simulink model "SimulacionCTRL3deposicion"  (R2021b)
settings: Solver=VariableStepAuto  StartTime=0.0  StopTime=20  RelTol=1e-3
undefined symbols (not defined in the file): coefDen, coefNum, kdr, ki, ki2, kp, kpr
libraries: simulink x1
settings Model: Creator=nicol  LastModifiedBy=CASA

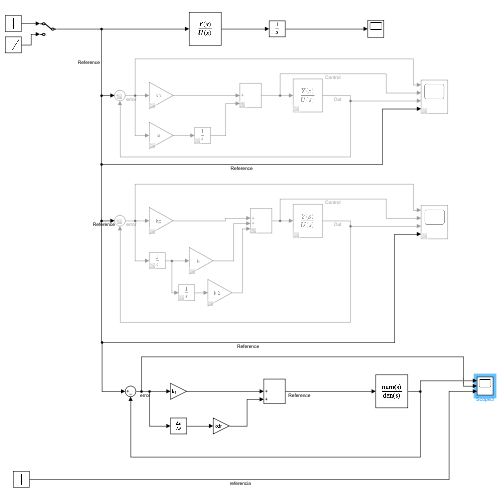
[thumbnail: Simulink's stored preview of the top-level diagram]
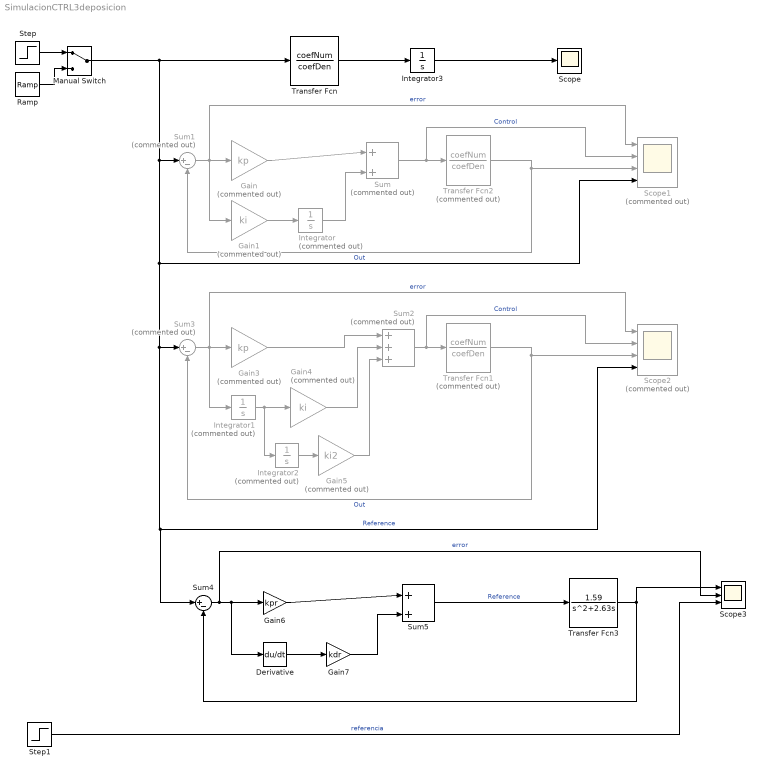
== system SimulacionCTRL3deposicion ==
  Derivative : Derivative
  Gain : Gain  Commented=on  Gain=kp
  Gain1 : Gain  Commented=on  Gain=ki
  Gain3 : Gain  Commented=on  Gain=kp
  Gain4 : Gain  Commented=on  Gain=ki
  Gain5 : Gain  Commented=on  Gain=ki2
  Gain6 : Gain  Gain=kpr
  Gain7 : Gain  Gain=kdr
  Integrator : Integrator  Commented=on
  Integrator1 : Integrator  Commented=on
  Integrator2 : Integrator  Commented=on
  Integrator3 : Integrator
  Manual Switch : ManualSwitch
  Ramp : simulink/Sources/Ramp  slope=1  start=0  InitialOutput=0
  Scope : Scope
  Scope1 : Scope  Commented=on  NumInputPorts=4
  Scope2 : Scope  Commented=on  NumInputPorts=4
  Scope3 : Scope  NumInputPorts=3
  Step : Step  Time=0  SampleTime=0
  Step1 : Step  Time=0  SampleTime=0
  Sum : Sum  Commented=on  Inputs=|++
  Sum1 : Sum  Commented=on  Inputs=|+-
  Sum2 : Sum  Commented=on  Inputs=|+++
  Sum3 : Sum  Commented=on  Inputs=|+-
  Sum4 : Sum  Inputs=|+-
  Sum5 : Sum  Inputs=|++
  Transfer Fcn : TransferFcn  Numerator=coefNum  Denominator=coefDen
  Transfer Fcn1 : TransferFcn  Commented=on  Numerator=coefNum  Denominator=coefDen
  Transfer Fcn2 : TransferFcn  Commented=on  Numerator=coefNum  Denominator=coefDen
  Transfer Fcn3 : TransferFcn  Numerator=[1.59]  Denominator=[1 2.63 0]
  wires:
  Gain1/1 -> Integrator/1
  Gain/1 -> Sum/1
  Integrator/1 -> Sum/2
  Sum/1 -> Scope1/2, Transfer Fcn2/1  "Control"
  Sum1/1 -> Gain1/1, Scope1/1, Gain/1  "error"
  Transfer Fcn2/1 -> Scope1/3, Sum1/2  "Out"
  Manual Switch/1 -> Sum3/1, Sum4/1, Scope2/4, Scope1/4, Sum1/1, Transfer Fcn/1  "Reference"
  Transfer Fcn1/1 -> Sum3/2, Scope2/3  "Out"
  Sum3/1 -> Gain3/1, Scope2/1, Integrator1/1  "error"
  Sum2/1 -> Transfer Fcn1/1, Scope2/2  "Control"
  Gain4/1 -> Sum2/2
  Gain3/1 -> Sum2/1
  Integrator1/1 -> Integrator2/1, Gain4/1
  Integrator2/1 -> Gain5/1
  Gain5/1 -> Sum2/3
  Step/1 -> Manual Switch/1
  Ramp/1 -> Manual Switch/2
  Transfer Fcn/1 -> Integrator3/1
  Integrator3/1 -> Scope/1
  Sum4/1 -> Scope3/2, Derivative/1, Gain6/1  "error"
  Derivative/1 -> Gain7/1
  Gain6/1 -> Sum5/1
  Gain7/1 -> Sum5/2
  Transfer Fcn3/1 -> Sum4/2, Scope3/1
  Sum5/1 -> Transfer Fcn3/1  "Reference"
  Step1/1 -> Scope3/3  "referencia"
